simulink model "FPGA_Comm_test_adc"  (Simulink 7.6)
settings: Solver=FixedStepDiscrete  StartTime=0.0  StopTime=500  FixedStep=0.01  MaxStep=1e-1  RelTol=1e-3
settings Model: Creator=jordan  LastModifiedBy=jordan
settings GRTTargetCC: ExtMode=on

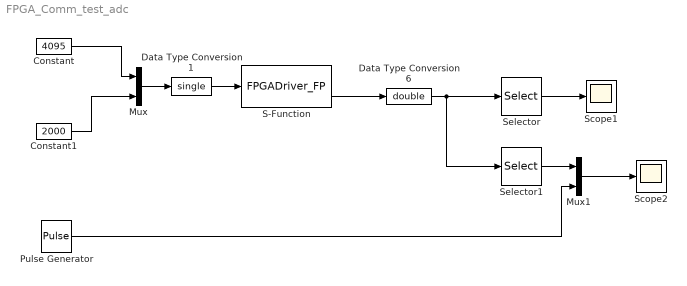
== system FPGA_Comm_test_adc ==
  Constant : Constant  Value=4095
  Constant1 : Constant  Value=2000
  Data Type Conversion1 : DataTypeConversion  OutDataTypeStr=single
  Data Type Conversion6 : DataTypeConversion  OutDataTypeStr=double
  Mux : Mux  Inputs=2
  Mux1 : Mux  Inputs=2
  Pulse Generator : DiscretePulseGenerator  Amplitude=2000  Period=100  PulseWidth=50  SampleTime=0.01
  S-Function : S-Function  FunctionName=FPGADriver_FP  EnableBusSupport=off
  Scope1 : Scope
      settings: TimeRange=50  YMin=0  YMax=4250  MaxDataPoints=50000
  Scope2 : Scope
      settings: TimeRange=50  YMin=0  YMax=4250  MaxDataPoints=50000
  Selector : Selector  InputPortWidth=2  IndexOptions=Index vector (dialog)  Indices=1  OutputSizes=1
  Selector1 : Selector  InputPortWidth=2  IndexOptions=Index vector (dialog)  Indices=2  OutputSizes=1
  wires:
  S-Function/2 -> Data Type Conversion6/1
  Data Type Conversion1/1 -> S-Function/1
  Data Type Conversion6/1 -> Selector/1, Selector1/1
  Mux/1 -> Data Type Conversion1/1
  Selector/1 -> Scope1/1
  Selector1/1 -> Mux1/1
  Constant/1 -> Mux/1
  Constant1/1 -> Mux/2
  Pulse Generator/1 -> Mux1/2
  Mux1/1 -> Scope2/1
